simulink model "Linealizacion"  (R2024a)
settings: Solver=VariableStepAuto  StartTime=0.0  StopTime=100  RelTol=1e-3
settings Model: Creator=alfre  LastModifiedBy=ansm3
settings RTWCC: GPUComputeCapability=3.5

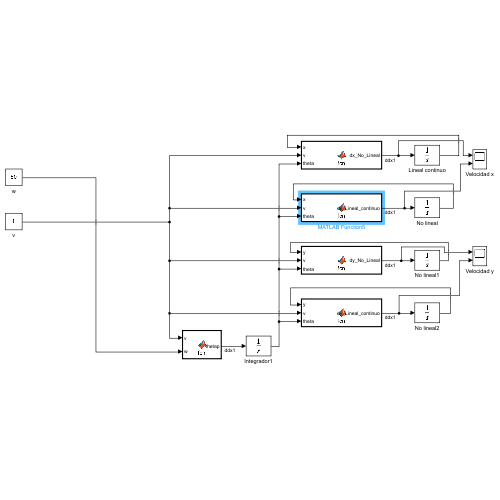
[thumbnail: Simulink's stored preview of the top-level diagram]
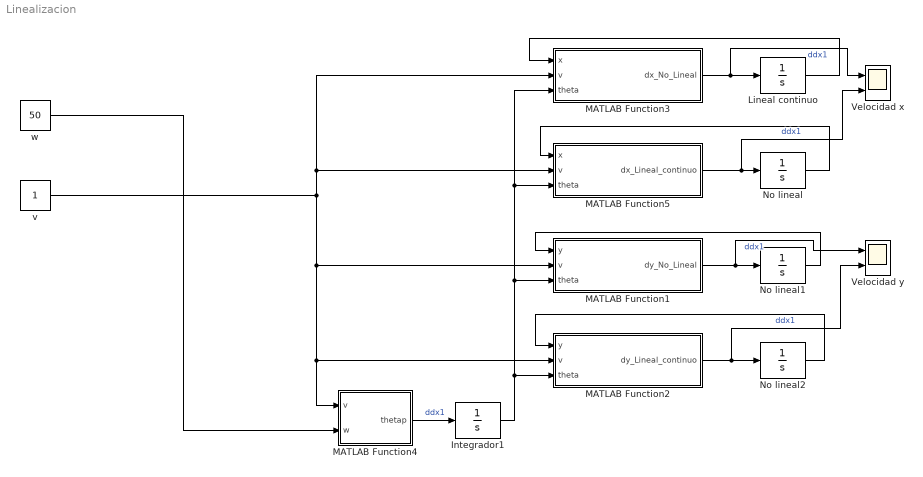
== system Linealizacion ==
  Integrador1 : Integrator  ContinuousStateAttributes="\"dx\""
  Lineal continuo : Integrator  ContinuousStateAttributes="\"dx\""
  MATLAB Function1 : MATLAB Function  TreatAsAtomicUnit=on
  MATLAB Function2 : MATLAB Function  TreatAsAtomicUnit=on
  MATLAB Function3 : MATLAB Function  TreatAsAtomicUnit=on
  MATLAB Function4 : MATLAB Function  TreatAsAtomicUnit=on
  MATLAB Function5 : MATLAB Function  TreatAsAtomicUnit=on
  No lineal : Integrator  ContinuousStateAttributes="\"dx\""
  No lineal1 : Integrator  ContinuousStateAttributes="\"dx\""
  No lineal2 : Integrator  ContinuousStateAttributes="\"dx\""
  Velocidad x : Scope  NumInputPorts=2
  Velocidad y : Scope  NumInputPorts=2
  v : Constant
  w : Constant  Value=50
  wires:
  Lineal continuo/1 -> MATLAB Function3/1(x)
  Integrador1/1 -> MATLAB Function2/3(theta), MATLAB Function1/3(theta), MATLAB Function5/3(theta), MATLAB Function3/3(theta)
  MATLAB Function3/1(dx_No_Lineal) -> Velocidad x/1, Lineal continuo/1  "ddx1"
  No lineal/1 -> MATLAB Function5/1(x)
  w/1 -> MATLAB Function4/2(w)
  MATLAB Function5/1(dx_Lineal_continuo) -> Velocidad x/2, No lineal/1  "ddx1"
  MATLAB Function4/1(thetap) -> Integrador1/1  "ddx1"
  v/1 -> MATLAB Function3/2(v), MATLAB Function5/2(v), MATLAB Function1/2(v), MATLAB Function4/1(v), MATLAB Function2/2(v)
  MATLAB Function1/1(dy_No_Lineal) -> Velocidad y/1, No lineal1/1  "ddx1"
  No lineal1/1 -> MATLAB Function1/1(y)
  MATLAB Function2/1(dy_Lineal_continuo) -> Velocidad y/2, No lineal2/1  "ddx1"
  No lineal2/1 -> MATLAB Function2/1(y)

== matlab function Linealizacion/MATLAB Function1 ==
  data: y input; v input; dy_No_Lineal output; theta input
function dy_No_Lineal = fcn(y, v, theta)
dy_No_Lineal= v*sin(theta);
dy_Lineal_continuo = v*cos(theta)*theta
dy_Lineal_discreto = y + v*cos(theta)*theta

== matlab function Linealizacion/MATLAB Function2 ==
  data: y input; v input; dy_Lineal_continuo output; theta input
function dy_Lineal_continuo = fcn(y, v, theta)
dx_No_Lineal= v*sin(theta);
dy_Lineal_continuo = v*cos(theta)*theta
dy_Lineal_discreto = y + v*cos(theta)*theta

== matlab function Linealizacion/MATLAB Function3 ==
  data: x input; v input; dx_No_Lineal output; theta input
function dx_No_Lineal = fcn(x, v, theta)
dx_No_Lineal= v*cos(theta);
dx_Lineal_continuo = -v*sin(theta)*theta
dx_Lineal_discreto = x -v*sin(theta)*theta

== matlab function Linealizacion/MATLAB Function4 ==
  data: v input; w input; thetap output
function thetap = fcn(v,w)
r=1;
w=v/r;
thetap=w;

== matlab function Linealizacion/MATLAB Function5 ==
  data: x input; v input; dx_Lineal_continuo output; theta input
function dx_Lineal_continuo = fcn(x, v, theta)
dx_No_Lineal= v*cos(theta);
dx_Lineal_continuo = -v*sin(theta)*theta
dx_Lineal_discreto = x -v*sin(theta)*theta
